simulink library "SimscapeCustomComponents_lib"  (R2025b)
settings: Solver=VariableStepAuto  StartTime=0.0  StopTime=10.0  RelTol=1e-3
undefined symbols (not defined in the file or in its folder): base, baseVdc, capacity, DiscIntNeverNeededParam, ee_sli_rtmsupport, filterInductance, freqeuncy, frequency, gcbh, gflInverter, gfmInverter, iMaxPU, Inertia, initialSOC, plantRating, solar, Ts, ups, Vac, windSystem, windTurbine
libraries: fl_lib x397, nesl_utility x171, eeGeneralControl x85, ee_lib x82, simulink x72, datacenter_lib x68, eeTransforms x38, slpidlib x24, buildingEnergy_lib x20, SimscapeFluids_lib x17, eeSinusoidalMeasurementV2 x8, eePwmGenerator x8
(part 21 of 24)

== system SimscapeCustomComponents_lib/Microgrid and Renewables/Sources/Solar Plant Integrated/Detailed/PV Plant & Controller/PV Plant/Converter/Switching ==
  mabc : Inport
  Add : Sum
  Constant1 : Constant
  Converter : ee_lib/Semiconductors & Converters/Converters/Converter (Three-Phase)  port_option=ee.enum.threePhasePort.composite  fidelity_option=ee.enum.converters.fidelity.detailed  device_type=ee.enum.converters.switchingdevice.ideal  showThermalPort=false  K=0  Vth=1 V  Vgt=1 V  Vgt_off=-1 V  Ih=1 A  Vf=0.8 V  Ron=0.001 Ohm  Rds=0.001 Ohm  Goff=1e-6 1/Ohm  Eon_scalar=22.86e-3 J  Eoff_scalar=17.14e-3 J  Eoff_natural_commutation=10e-3 J  Voff=300 V  Iout_scalar=600 A  onCurrentMeasDelay=0 s  useCurrentFromPreviousCycle=false  useVoltageFromPreviousCycle=false  diode_param=ee.enum.converters.protectiondiode.nodynamics  diode_Vf=0.01 V  diode_Ron=0.0001 Ohm  diode_Goff=1e-5 1/Ohm  diode_C=50 nF  diode_iRM=-235 A  diode_iF=300 A  diode_idot=-50 A/us  diode_trr_param=ee.enum.converters.diodetrr.trr_factor  diode_trr_factor=3  diode_trr=15 us  diode_Qrr=1500 s*uA  diode_rec_loss_model=ee.enum.diode.reverseRecoveryModel.fixed  diode_ErecVal=0 J  diode_scaleWithIandV=false  diode_ErecMat=zeros(2, 3) J  diode_TjrecVec=[298.15, 398.15] K  diode_IfrecVec=[.1, 1, 10] A  diode_IrecVal=10 A  diode_VrecVal=10 V  diode_tFilter=1 / 1000 / 100 s  thermal_network_parameterization=ee.enum.thermalNetworkTopology.external  Rth=[.08, .5] K/W  Rth_Cauer=[.08, .1, .5] K/W  Rth_Foster=[.08, .14, .22, .16] K/W  thermal_mass_parameterization=ee.enum.thermalNetwork.timeconstant  thermal_mass=[.01, .5] J/K  thermal_mass_Cauer=[.01, .1, .5] J/K  thermal_mass_Foster=[.001, .005, .05, .5] J/K  thermal_time_constant=[.001, .2] s  thermal_time_constant_Cauer=[.001, .1, .2] s  thermal_time_constant_Foster=[7e-05, .0007, .01, .08] s  thermal_mass_initial_temperatures=[25, 25] degC  thermal_mass_initial_temperatures_Cauer=[25, 25, 25] degC  junction_thermal_mass=0.01 J/K  Tvec_initial_Foster=[25, 25, 25, 25] degC  snubber_type=ee.enum.converters.snubber.exclude  Cs=1e-7 F  Rs=0.1 Ohm  Vce_loss=[0, 150, 300] V
  Demux : Demux  Outputs=3
  Demux1 : Demux  Outputs=3
  Gain : Gain  Gain=5
  Gain1 : Gain  Gain=0.5
  PWM Generator : eePwmGenerator/PWM Generator  CarrCount=Up  Tper=1/(fSw*1000)  Tdelay=0  Ts=1/(10*fSw*1000)
  Pulse Generation : Subsystem
  Rate Transition1 : RateTransition  OutPortSampleTime=1/(10*fSw*1000)
  Simulink-PS Converter{1..6} (6 alike) : nesl_utility/Simulink-PS Converter  PhysicalDomain=network_engine_domain  SubClassName=ps_input  LeftPortType=input  RightPortType=output  PseudoPeriodic=off  Frequencies=[]  NoiseDistribution=none  NoiseParameters=[]  Unit=1  AffineConversion=off  FilteringAndDerivatives=provide  SimscapeFilterOrder=1  InputFilterTimeConstant=0.001  UdotUserProvided=0
  Six-Pulse Gate Multiplexer : ee_lib/Semiconductors & Converters/Converters/Six-Pulse Gate Multiplexer  port_option=ee.enum.controlport.ps
  + : PMIOPort  Side=Left
  ~ : PMIOPort  Port=2  Side=Right
  - : PMIOPort  Port=3  Side=Left
  wires:
  [BH] -> Simulink-PS Converter4/1
  Pulse Generation/1(G1) -> Demux/1
  Pulse Generation/2(G2) -> Demux1/1
  Rate Transition1/1 -> PWM Generator/1
  Demux/1 -> [AH]
  Demux1/2 -> [BL]
  [AL] -> Simulink-PS Converter5/1
  [CH] -> Simulink-PS Converter2/1
  mabc/1 -> Add/1
  PWM Generator/1 -> Gain/1
  Gain/1 -> Pulse Generation/1(G)
  Add/1 -> Gain1/1
  Constant1/1 -> Add/2
  [CL] -> Simulink-PS Converter1/1
  Demux/2 -> [BH]
  Demux/3 -> [CH]
  Gain1/1 -> Rate Transition1/1
  Demux1/3 -> [CL]
  [AH] -> Simulink-PS Converter6/1
  [BL] -> Simulink-PS Converter3/1
  Demux1/1 -> [AL]
  connections:
  -/RConn1 -- Converter/RConn2
  +/RConn1 -- Converter/RConn1
  Six-Pulse Gate Multiplexer/LConn4 -- Simulink-PS Converter3/RConn1
  Six-Pulse Gate Multiplexer/LConn1 -- Simulink-PS Converter6/RConn1
  Six-Pulse Gate Multiplexer/RConn1 -- Converter/LConn1
  Six-Pulse Gate Multiplexer/LConn3 -- Simulink-PS Converter4/RConn1
  Simulink-PS Converter1/RConn1 -- Six-Pulse Gate Multiplexer/LConn6
  Simulink-PS Converter2/RConn1 -- Six-Pulse Gate Multiplexer/LConn5
  Six-Pulse Gate Multiplexer/LConn2 -- Simulink-PS Converter5/RConn1
  ~/RConn1 -- Converter/LConn2

== system SimscapeCustomComponents_lib/Microgrid and Renewables/Sources/Wind Plant Integrated/Detailed/Wind Turbine and Converters/Wind Controller/Machine Converter Control/Measurements ==
  iabc_sens : Inport
  w_sens : Inport  Port=2
  th_sens : Inport  Port=3
  Vdc_sens : Inport  Port=4
  2*pi : Constant  Value=2*pi  SampleTime=-1
  Math Function : Math  Operator=mod  SignedPower=on
  pole pairs : Gain  Gain=p
  "pole pairs " : Gain  Gain=p
  we : Outport  VectorParamsAs1DForOutWhenUnconnected=off
  iabc : Outport  Port=2  VectorParamsAs1DForOutWhenUnconnected=off
  theta : Outport  Port=3  VectorParamsAs1DForOutWhenUnconnected=off
  Vdc : Outport  Port=4  VectorParamsAs1DForOutWhenUnconnected=off
  wires:
  w_sens/1 -> pole pairs/1
  iabc_sens/1 -> iabc/1
  pole pairs/1 -> we/1
  2*pi/1 -> Math Function/2
  th_sens/1 -> "pole pairs "/1
  "pole pairs "/1 -> Math Function/1
  Vdc_sens/1 -> Vdc/1
  Math Function/1 -> theta/1

== system SimscapeCustomComponents_lib/Microgrid and Renewables/Sources/Wind Plant Integrated/Detailed/Wind Turbine and Converters/Wind Controller/Machine Converter Control/Power Controller ==
  windSpeed : Inport
  Derating Control : Subsystem
  Greater than : simulink/Logic and Bit Operations/Compare To Constant  relop=>  const=12  OutDataTypeStr=boolean
  Less than or equal to : simulink/Logic and Bit Operations/Compare To Constant  relop=<=  const=12  OutDataTypeStr=boolean
  Limiter Function Power Demand : Subsystem
  MPPT Control : Subsystem
  activePowerDemand : Outport
  wires:
  windSpeed/1 -> Greater than/1, Less than or equal to/1, MPPT Control/1(windSpeed)
  Less than or equal to/1 -> MPPT Control/Enable
  Greater than/1 -> Derating Control/Enable
  MPPT Control/1(activePowerDemand) -> Limiter Function Power Demand/1(activePowerDemandMPPT)
  Derating Control/1(activePowerDemand) -> Limiter Function Power Demand/2(activePowerDemandDerating)
  Limiter Function Power Demand/1(activePowerDemand) -> activePowerDemand/1

== system SimscapeCustomComponents_lib/Microgrid and Renewables/Sources/Wind Plant Integrated/Detailed/Wind Turbine and Converters/Wind Controller/Machine Converter Control/Subsystem ==
  note: LVRT Crowbar Control
  Vdc : Inport
  LVRT : Inport  Port=2
  Abs : Abs  SaturateOnIntegerOverflow=off
  Constant1 : Constant  Value=Vdc
  Product : Product
  Relay : Relay  OnSwitchValue=0.01001*Vdc  OffSwitchValue=0.01*Vdc
  Sum : Sum  Inputs=|+-
  Unit Delay1 : UnitDelay  SampleTime=-1
  Out1 : Outport
  wires:
  Constant1/1 -> Sum/1
  Vdc/1 -> Unit Delay1/1
  Sum/1 -> Product/1
  Abs/1 -> Relay/1
  Unit Delay1/1 -> Sum/2
  LVRT/1 -> Product/2
  Product/1 -> Abs/1
  Relay/1 -> Out1/1

== system SimscapeCustomComponents_lib/Microgrid and Renewables/Sources/Wind Plant Integrated/Detailed/Wind Turbine and Converters/Wind Controller/Wind Grid-side Converter Controller/Current_controller ==
  iWindd : Inport
  iq : Inport  Port=2
  id-ref : Inport  Port=3
  iqref : Inport  Port=4
  Vd : Inport  Port=5
  Vq : Inport  Port=6
  Constant4 : Constant  Value=0
  Gain1 : Gain  Gain=2*1*pi*frequency*inductance/baseImpedance
  Gain2 : Gain  Gain=2*1*pi*frequency*inductance/baseImpedance
  Mux1 : Mux  Inputs=3
  PI : Subsystem
  PI1 : Subsystem
  Sum1 : Sum  Inputs=|+-
  Sum3 : Sum  Inputs=|++-
  Sum4 : Sum  Inputs=|+++
  Sum5 : Sum  Inputs=|+-
  Refrence_mdq0 : Outport
  wires:
  PI/1(Out2) -> Sum3/2
  Sum3/1 -> Mux1/1, [Ed]
  Gain2/1 -> Sum3/3
  iWindd/1 -> Gain1/1, Sum1/2
  id-ref/1 -> Sum1/1
  Gain1/1 -> Sum4/3
  Vq/1 -> Sum4/2
  iq/1 -> Gain2/1, Sum5/2
  Sum1/1 -> PI/1(Input)
  Vd/1 -> Sum3/1
  Constant4/1 -> Mux1/3
  Sum5/1 -> PI1/1(Input)
  iqref/1 -> Sum5/1
  PI1/1(Out2) -> Sum4/1
  Sum4/1 -> Mux1/2, [Eq]
  Mux1/1 -> Refrence_mdq0/1  "m_dqo"

== system SimscapeCustomComponents_lib/Microgrid and Renewables/Sources/Wind Plant Integrated/Detailed/Wind Turbine and Converters/Wind Controller/Wind Grid-side Converter Controller/DC Bus Chopper control  ==
  note: LVRT Detection
  In1 : Inport
  Constant1 : Constant
  Constant2 : Constant  Value=0
  Switch : Switch  Criteria=u2 > Threshold  Threshold=0.9  SaturateOnIntegerOverflow=off  InputSameDT=off
  Unit Delay : UnitDelay  SampleTime=-1
  Out1 : Outport
  wires:
  Switch/1 -> Out1/1
  Constant1/1 -> Switch/3
  Constant2/1 -> Switch/1
  In1/1 -> Unit Delay/1
  Unit Delay/1 -> Switch/2

== system SimscapeCustomComponents_lib/Microgrid and Renewables/Sources/Wind Plant Integrated/Detailed/Wind Turbine and Converters/Wind Controller/Wind Grid-side Converter Controller/DC voltage controller & current reference ==
  note: Limiter
  note: iq_ref_generator
  note: id_ref_generator
  Q_ref : Inport
  Vmag : Inport  Port=2
  Wind_Mpp_vdc : Inport  Port=3
  Wind_vdc : Inport  Port=4
  lvrt.iq : Inport  Port=5
  Constant : Constant
  Constant1 : Constant  Value=iMaxPU
  Current limits : Subsystem
  Subsystem : Subsystem
  Subsystem1 : Subsystem
  Switch : Switch  Criteria=u2 > Threshold  SaturateOnIntegerOverflow=off  InputSameDT=off
  Unit Delay1 : UnitDelay  SampleTime=Ts
  Unit Delay3 : UnitDelay  SampleTime=Ts
  id_ref : Outport
  iq_ref : Outport  Port=2
  wires:
  Current limits/2(iubd) -> Subsystem1/3(id_ub)
  Subsystem/1(Out1) -> Unit Delay1/1, iq_ref/1
  Constant1/1 -> Current limits/1(Imax)
  Unit Delay1/1 -> Current limits/2(iqref)
  Subsystem1/1(Out1) -> id_ref/1, Unit Delay3/1
  Unit Delay3/1 -> Current limits/3(idref)
  Q_ref/1 -> Subsystem/4(Q_ref)
  Wind_Mpp_vdc/1 -> Subsystem1/1(Wind_Mpp_vdc)
  Wind_vdc/1 -> Subsystem1/2(Wind_vdc)
  Current limits/1(iubq) -> Subsystem/2(iq_ub)
  lvrt.iq/1 -> Subsystem/3(lvrt.iq)
  Vmag/1 -> Switch/1, Switch/2
  Switch/1 -> Subsystem/1(V_mag)
  Constant/1 -> Switch/3

== system SimscapeCustomComponents_lib/Microgrid and Renewables/Sources/Wind Plant Integrated/Detailed/Wind Turbine and Converters/Wind Plant/Back-to-Back Converters/Average ==
  Chopper : Inport
  SM_ref : Inport  Port=2
  Grid_ref : Inport  Port=3
  Capacitor : fl_lib/Electrical/Electrical Elements/Capacitor  c=capDC F  r=1e-1 Ohm  g=0 1/Ohm  i_specify=off  i_priority=None  i=0 A  i_nominal_specify=off  i_nominal_value=1  i_nominal_unit=A  v_specify=off  v_priority=None  v=0 V  v_nominal_specify=off  v_nominal_value=1  v_nominal_unit=V  vc_specify=on  vc_priority=High  vc=Vdc V  vc_nominal_specify=off  vc_nominal_value=1  vc_nominal_unit=V
  Electrical Reference : fl_lib/Electrical/Electrical Elements/Electrical Reference
  Electrical Reference1 : fl_lib/Electrical/Electrical Elements/Electrical Reference
  Electrical Reference2 : fl_lib/Electrical/Electrical Elements/Electrical Reference
  Grid Side Converter : ee_lib/Semiconductors & Converters/Converters/Average-Value Voltage Source Converter (Three-Phase)  port_option=ee.enum.threePhasePort.composite  frequency_option=ee.enum.converters.frequency.variable  input_option=ee.enum.converters.inputOption.ModWave  FRated=60 Hz  losses_parameterization=ee.enum.converters.losses.fixed  Pfixed=1 W  ks=0.01  kc1=1.7 V  kc2=0.01 Ohm  Ploss_vect=[100, 800, 1870, 3250, 4900] W  Irms_vect=[10, 100, 200, 300, 400] A  Vdc_nom=300 V  thermal_mass=30000 J/K  temperature_specify=off  temperature_priority=High  temperature=298.15 K  temperature_nominal_specify=off  temperature_nominal_value=1  temperature_nominal_unit=K
      settings: InternalSimscapePortConfiguration="{\"Bottom\":[],\"Left\":[{\"id\":\"ModWave\",\"label\":\"ModWave\",\"type\":\"input\"},{\"id\":\"N\",\"label\":\"~\",\"type\":\"foundation.electrical.three_phase\"}],\"Right\":[{\"id\":\"p\",\"label\":\"+\",\"type\":\"foundation.electrical.electrical\"},{\"id\":\"n\",\"label\":\"-\",\"type\":\"foundation.electrical.electrical\"}],\"Top\":[]}"
  Ideal Semiconductor Switch : ee_lib/Semiconductors & Converters/Ideal Semiconductor Switch  port_option=ee.enum.controlport.ps  Ron=0.001 Ohm  Goff=1e-6 1/Ohm  Vth=0.5 V  diode_param=ee.enum.converters.protectiondiode.none  diode_Vf=0.8 V  diode_Ron=0.001 Ohm  diode_Goff=1e-5 1/Ohm  diode_C=50e-9 F  diode_iRM=-235 A  diode_iF=300 A  diode_idot=-50 A/us  diode_trr_param=ee.enum.converters.diodetrr.trr_factor  diode_trr_factor=3  diode_trr=15 us  diode_Qrr=1500 s*uA
  Machine Side Converter : ee_lib/Semiconductors & Converters/Converters/Average-Value Voltage Source Converter (Three-Phase)  port_option=ee.enum.threePhasePort.composite  frequency_option=ee.enum.converters.frequency.variable  input_option=ee.enum.converters.inputOption.ModWave  FRated=60 Hz  losses_parameterization=ee.enum.converters.losses.fixed  Pfixed=1 W  ks=0.01  kc1=1.7 V  kc2=0.01 Ohm  Ploss_vect=[100, 800, 1870, 3250, 4900] W  Irms_vect=[10, 100, 200, 300, 400] A  Vdc_nom=300 V  thermal_mass=30000 J/K  temperature_specify=off  temperature_priority=High  temperature=298.15 K  temperature_nominal_specify=off  temperature_nominal_value=1  temperature_nominal_unit=K
      settings: InternalSimscapePortConfiguration="{\"Bottom\":[],\"Left\":[{\"id\":\"ModWave\",\"label\":\"ModWave\",\"type\":\"input\"},{\"id\":\"N\",\"label\":\"~\",\"type\":\"foundation.electrical.three_phase\"}],\"Right\":[{\"id\":\"p\",\"label\":\"+\",\"type\":\"foundation.electrical.electrical\"},{\"id\":\"n\",\"label\":\"-\",\"type\":\"foundation.electrical.electrical\"}],\"Top\":[]}"
  PS-Simulink Converter1 : nesl_utility/PS-Simulink Converter  PhysicalDomain=network_engine_domain  SubClassName=ps_output  LeftPortType=input  RightPortType=output  PseudoPeriodic=off  Frequencies=[]  VectorFormat=1-D array  Unit=V  AffineConversion=off
  Resistor : fl_lib/Electrical/Electrical Elements/Resistor  R=16 Ohm  i_specify=off  i_priority=None  i=0 A  i_nominal_specify=off  i_nominal_value=1  i_nominal_unit=A  v_specify=off  v_priority=None  v=0 V  v_nominal_specify=off  v_nominal_value=1  v_nominal_unit=V
  Scope : Scope
      settings: ActiveDisplayYMinimum=-0.125  ActiveDisplayYMaximum=1.125  DataLoggingVariableName=ScopeData11
  Simulink-PS Converter : nesl_utility/Simulink-PS Converter  PhysicalDomain=network_engine_domain  SubClassName=ps_input  LeftPortType=input  RightPortType=output  PseudoPeriodic=off  Frequencies=[]  NoiseDistribution=none  NoiseParameters=[]  Unit=1  AffineConversion=off  FilteringAndDerivatives=provide  SimscapeFilterOrder=1  InputFilterTimeConstant=0.001  UdotUserProvided=0
  Simulink-PS Converter2 : nesl_utility/Simulink-PS Converter  PhysicalDomain=network_engine_domain  SubClassName=ps_input  LeftPortType=input  RightPortType=output  PseudoPeriodic=off  Frequencies=[]  NoiseDistribution=none  NoiseParameters=[]  Unit=1  AffineConversion=off  FilteringAndDerivatives=provide  SimscapeFilterOrder=1  InputFilterTimeConstant=0.001  UdotUserProvided=0
  Simulink-PS Converter4 : nesl_utility/Simulink-PS Converter  PhysicalDomain=network_engine_domain  SubClassName=ps_input  LeftPortType=input  RightPortType=output  PseudoPeriodic=off  Frequencies=[]  NoiseDistribution=none  NoiseParameters=[]  Unit=1  AffineConversion=off  FilteringAndDerivatives=provide  SimscapeFilterOrder=1  InputFilterTimeConstant=0.001  UdotUserProvided=0
  Voltage Sensor : fl_lib/Electrical/Electrical Sensors/Voltage Sensor
  In : PMIOPort  Side=Left
  ~ : PMIOPort  Port=2  Side=Right
  Vdc : Outport
  wires:
  Grid_ref/1 -> Simulink-PS Converter4/1
  Chopper/1 -> Scope/1, Simulink-PS Converter2/1
  PS-Simulink Converter1/1 -> Vdc/1  "Vdc"
  SM_ref/1 -> Simulink-PS Converter/1
  connections:
  Electrical Reference/LConn1 -- Machine Side Converter/RConn2 -- Voltage Sensor/RConn2 -- Capacitor/RConn1
  Grid Side Converter/RConn1 -- Ideal Semiconductor Switch/RConn1 -- Capacitor/LConn1 -- Machine Side Converter/RConn1 -- Voltage Sensor/LConn1
  Electrical Reference2/LConn1 -- Grid Side Converter/RConn2
  PS-Simulink Converter1/LConn1 -- Voltage Sensor/RConn1
  ~/RConn1 -- Grid Side Converter/LConn2
  Resistor/LConn1 -- Ideal Semiconductor Switch/RConn2
  Grid Side Converter/LConn1 -- Simulink-PS Converter4/RConn1
  Electrical Reference1/LConn1 -- Resistor/RConn1
  Simulink-PS Converter2/RConn1 -- Ideal Semiconductor Switch/LConn1
  Machine Side Converter/LConn2 -- In/RConn1
  Simulink-PS Converter/RConn1 -- Machine Side Converter/LConn1

== system SimscapeCustomComponents_lib/Microgrid and Renewables/Sources/Wind Plant Integrated/Detailed/Wind Turbine and Converters/Wind Plant/Back-to-Back Converters/Switching ==
  Chopper : Inport
  SM_ref : Inport  Port=2
  Grid_ref : Inport  Port=3
  Capacitor : fl_lib/Electrical/Electrical Elements/Capacitor  c=capacitance F  r=1e-1 Ohm  g=0 1/Ohm  i_specify=off  i_priority=None  i=0 A  i_nominal_specify=off  i_nominal_value=1  i_nominal_unit=A  v_specify=off  v_priority=None  v=0 V  v_nominal_specify=off  v_nominal_value=1  v_nominal_unit=V  vc_specify=on  vc_priority=High  vc=baseVoltageDC V  vc_nominal_specify=off  vc_nominal_value=1  vc_nominal_unit=V
  Electrical Reference : fl_lib/Electrical/Electrical Elements/Electrical Reference
  Electrical Reference1 : fl_lib/Electrical/Electrical Elements/Electrical Reference
  Electrical Reference2 : fl_lib/Electrical/Electrical Elements/Electrical Reference
  Grid Side Converter : Subsystem
      settings: PortSchema="{\"entries\":[{\"content\":{\"sides\":[{\"content\":{\"connectorIds\":[\"LConn1\",\"LConn2\"]},\"type\":\"ConnectorPlacement.EquallySpacedRectSide\",\"uuid\":\"e32be008-cebd-46aa-ba62-c5c92b9b23e3\"},{\"content\":{\"connectorIds\":[\"In1\",\"RConn1\"],\"side\":\"RIGHT\"},\"type\":\"ConnectorPlacement.EquallySpacedRectSide\",\"uuid\":\"c483e451-04b5-4212-bdd1-c589ba5bea78\"},{\"content\":{\"side\":\"TOP\"},\"type\":\"ConnectorPlacement.EquallySpacedRectSide\",\"uuid\":\"824c135c-7e5f-4da0-a7de-e626b4bfa50d\"}]},\"type\":\"ConnectorPlacement.EquallySpacedConnector\",\"uuid\":\"5f81c72d-92ab-4525-91a6-193f769a7c86\"}],\"packageUris\":[\"http://schema.mathworks.com/mf0/Connector/R2020b\"],\"version\":\"1.0\"}"
  Ideal Semiconductor Switch : ee_lib/Semiconductors & Converters/Ideal Semiconductor Switch  port_option=ee.enum.controlport.ps  Ron=0.001 Ohm  Goff=1e-6 1/Ohm  Vth=0.5 V  diode_param=ee.enum.converters.protectiondiode.none  diode_Vf=0.8 V  diode_Ron=0.001 Ohm  diode_Goff=1e-5 1/Ohm  diode_C=50e-9 F  diode_iRM=-235 A  diode_iF=300 A  diode_idot=-50 A/us  diode_trr_param=ee.enum.converters.diodetrr.trr_factor  diode_trr_factor=3  diode_trr=15 us  diode_Qrr=1500 s*uA
  Machine Side Converter : Subsystem
      settings: PortSchema="{\"entries\":[{\"content\":{\"sides\":[{\"content\":{\"connectorIds\":[\"LConn1\",\"LConn2\"]},\"type\":\"ConnectorPlacement.EquallySpacedRectSide\",\"uuid\":\"e32be008-cebd-46aa-ba62-c5c92b9b23e3\"},{\"content\":{\"connectorIds\":[\"In1\",\"RConn1\"],\"side\":\"RIGHT\"},\"type\":\"ConnectorPlacement.EquallySpacedRectSide\",\"uuid\":\"c483e451-04b5-4212-bdd1-c589ba5bea78\"},{\"content\":{\"side\":\"TOP\"},\"type\":\"ConnectorPlacement.EquallySpacedRectSide\",\"uuid\":\"824c135c-7e5f-4da0-a7de-e626b4bfa50d\"}]},\"type\":\"ConnectorPlacement.EquallySpacedConnector\",\"uuid\":\"5f81c72d-92ab-4525-91a6-193f769a7c86\"}],\"packageUris\":[\"http://schema.mathworks.com/mf0/Connector/R2020b\"],\"version\":\"1.0\"}"
  PS-Simulink Converter1 : nesl_utility/PS-Simulink Converter  PhysicalDomain=network_engine_domain  SubClassName=ps_output  LeftPortType=input  RightPortType=output  PseudoPeriodic=off  Frequencies=[]  VectorFormat=1-D array  Unit=V  AffineConversion=off
  Resistor : fl_lib/Electrical/Electrical Elements/Resistor  R=16 Ohm  i_specify=off  i_priority=None  i=0 A  i_nominal_specify=off  i_nominal_value=1  i_nominal_unit=A  v_specify=off  v_priority=None  v=0 V  v_nominal_specify=off  v_nominal_value=1  v_nominal_unit=V
  Scope : Scope
      settings: ActiveDisplayYMinimum=-0.125  ActiveDisplayYMaximum=1.125  DataLoggingVariableName=ScopeData11
  Simulink-PS Converter2 : nesl_utility/Simulink-PS Converter  PhysicalDomain=network_engine_domain  SubClassName=ps_input  LeftPortType=input  RightPortType=output  PseudoPeriodic=off  Frequencies=[]  NoiseDistribution=none  NoiseParameters=[]  Unit=1  AffineConversion=off  FilteringAndDerivatives=provide  SimscapeFilterOrder=1  InputFilterTimeConstant=0.001  UdotUserProvided=0
  Voltage Sensor : fl_lib/Electrical/Electrical Sensors/Voltage Sensor
  In : PMIOPort  Side=Left
  ~ : PMIOPort  Port=2  Side=Right
  Vdc : Outport
  wires:
  SM_ref/1 -> Machine Side Converter/1(mabc)
  Grid_ref/1 -> Grid Side Converter/1(mabc)
  Chopper/1 -> Scope/1, Simulink-PS Converter2/1
  PS-Simulink Converter1/1 -> Vdc/1  "Vdc"
  connections:
  Machine Side Converter/LConn2 -- Voltage Sensor/RConn2 -- Capacitor/RConn1 -- Electrical Reference/LConn1
  Ideal Semiconductor Switch/RConn1 -- Grid Side Converter/LConn1 -- Capacitor/LConn1 -- Machine Side Converter/LConn1 -- Voltage Sensor/LConn1
  Grid Side Converter/LConn2 -- Electrical Reference2/LConn1
  PS-Simulink Converter1/LConn1 -- Voltage Sensor/RConn1
  ~/RConn1 -- Grid Side Converter/RConn1
  Resistor/LConn1 -- Ideal Semiconductor Switch/RConn2
  Electrical Reference1/LConn1 -- Resistor/RConn1
  Simulink-PS Converter2/RConn1 -- Ideal Semiconductor Switch/LConn1
  Machine Side Converter/RConn1 -- In/RConn1

== system SimscapeCustomComponents_lib/Microgrid and Renewables/Storage/BESS Integrated/Detailed/BESS Controller/Grid Following/Reference Current/Current limits ==
  Imax : Inport
  iqref : Inport  Port=2
  idref : Inport  Port=3
  Constant8 : Constant  Value=0
  Constant9 : Constant  Value=0
  Scope : Scope
      settings: ActiveDisplayYMinimum=-0.14399  ActiveDisplayYMaximum=1.29587  DataLoggingVariableName=ScopeData3
  Scope1 : Scope
      settings: ActiveDisplayYMinimum=-0.13655  ActiveDisplayYMaximum=1.22893  DataLoggingVariableName=ScopeData4
  Sqrt : Sqrt
  Sqrt1 : Sqrt
  Square{1..4} (4 alike) : Math  Operator=square
  Step2 : Step  Time=0.01  SampleTime=Ts
  Step3 : Step  Time=0.01  SampleTime=Ts
  Sum6 : Sum  Inputs=|+-
  Sum9 : Sum  Inputs=|+-
  Switch1 : Switch  Threshold=.01  SaturateOnIntegerOverflow=off  InputSameDT=off
  Switch2 : Switch  Threshold=.01  SaturateOnIntegerOverflow=off  InputSameDT=off
  iubq : Outport
  iubd : Outport  Port=2
  wires:
  Sum9/1 -> Switch2/1
  Step3/1 -> Switch2/2
  Step2/1 -> Switch1/2
  Switch2/1 -> Sqrt1/1
  Square1/1 -> Sum6/1
  Switch1/1 -> Sqrt/1
  iqref/1 -> Square2/1
  Square3/1 -> Sum9/1
  Sum6/1 -> Switch1/1
  Square2/1 -> Sum6/2
  Constant8/1 -> Switch1/3
  Square4/1 -> Sum9/2
  Constant9/1 -> Switch2/3
  Sqrt/1 -> Scope/1, iubd/1
  Imax/1 -> Square3/1, Square1/1
  Sqrt1/1 -> Scope1/1, iubq/1
  idref/1 -> Square4/1

== system SimscapeCustomComponents_lib/Microgrid and Renewables/Storage/BESS Integrated/Detailed/BESS Controller/Grid Following/Reference Current/Refernce id generation ==
  V_mag : Inport
  del f : Inport  Port=2
  ubid : Inport  Port=3
  PRef : Inport  Port=4
  Divide : Product  Inputs=/*
  Gain6 : Gain  Gain=-1
  P/Q Priority : Switch  Criteria=u2 ~= 0  SaturateOnIntegerOverflow=off  InputSameDT=off
  Priority Mode : Constant  Value=P-2
  Saturation Dynamic2 : simulink/Discontinuities/Saturation Dynamic  OutMin=[]  OutMax=[]  OutDataTypeStr=Inherit: Same as second input  OutDataType=fixdt(1, 16)  OutScaling=2^-10  DoSatur=off
  Saturation1 : Saturate  UpperLimit=Imax  LowerLimit=-Imax
  Scope : Scope
      settings: ActiveDisplayYMinimum=-1  ActiveDisplayYMaximum=1
  Scope1 : Scope
      settings: ActiveDisplayYMinimum=-0.68622  ActiveDisplayYMaximum=0.07625  DataLoggingVariableName=ScopeData2
  Sum : Sum  Inputs=|++
  droop m_p : Gain  Gain=mp/MVA
  ubid1 : InportShadow  Port=3
  id_ref : Outport
  wires:
  droop m_p/1 -> Sum/1
  Sum/1 -> Divide/2
  ubid/1 -> Saturation Dynamic2/1
  Gain6/1 -> Saturation Dynamic2/3
  Saturation Dynamic2/1 -> Scope1/1, P/Q Priority/3
  PRef/1 -> Sum/2
  Priority Mode/1 -> P/Q Priority/2
  Saturation1/1 -> P/Q Priority/1
  ubid1/1 -> Gain6/1
  P/Q Priority/1 -> Scope/1, id_ref/1
  V_mag/1 -> Divide/1
  Divide/1 -> Saturation1/1, Saturation Dynamic2/2
  del f/1 -> droop m_p/1

== system SimscapeCustomComponents_lib/Microgrid and Renewables/Storage/BESS Integrated/Detailed/BESS Controller/Grid Following/Reference Current/Refernce iq generation ==
  ubiq : Inport
  V_ref : Inport  Port=2
  V_mag : Inport  Port=3
  LVRT_iq : Inport  Port=4
  Q_ref : Inport  Port=5
  Divide1 : Product  Inputs=*/
  Gain : Gain  Gain=-1
  Gain1 : Gain  Gain=-1
  Gain7 : Gain  Gain=-1
  LVRT Priority : Switch  Threshold=.9  SaturateOnIntegerOverflow=off  InputSameDT=off
  P/Q Priority : Switch  Criteria=u2 ~= 0  SaturateOnIntegerOverflow=off  InputSameDT=off
  Priority Mode : Constant  Value=P-2
  Saturation Dynamic : simulink/Discontinuities/Saturation Dynamic  OutMin=[]  OutMax=[]  OutDataTypeStr=Inherit: Same as second input  OutDataType=fixdt(1, 16)  OutScaling=2^-10  DoSatur=off
  Saturation2 : Saturate  UpperLimit=1  LowerLimit=-1
  Saturation3 : Saturate  UpperLimit=Imax  LowerLimit=-Imax
  Sum : Sum  Inputs=|++
  Sum1 : Sum  Inputs=|-+
  droop m_v : Gain  Gain=mv
  ubiq1 : InportShadow
  iq_ref : Outport
  wires:
  LVRT Priority/1 -> Gain/1
  Sum1/1 -> droop m_v/1
  P/Q Priority/1 -> LVRT Priority/1
  Gain1/1 -> LVRT Priority/3
  ubiq/1 -> Saturation Dynamic/1
  Saturation2/1 -> Gain1/1
  Saturation3/1 -> P/Q Priority/3
  Priority Mode/1 -> P/Q Priority/2
  Divide1/1 -> Saturation Dynamic/2, Saturation3/1
  Saturation Dynamic/1 -> P/Q Priority/1
  Gain7/1 -> Saturation Dynamic/3
  V_ref/1 -> Sum1/1
  LVRT_iq/1 -> Saturation2/1
  ubiq1/1 -> Gain7/1
  droop m_v/1 -> Sum/2
  Sum/1 -> Divide1/1
  Q_ref/1 -> Sum/1
  V_mag/1 -> LVRT Priority/2, Divide1/2, Sum1/2
  Gain/1 -> iq_ref/1

== system SimscapeCustomComponents_lib/Microgrid and Renewables/Storage/BESS Integrated/Detailed/BESS Controller/Grid Forming/Current Limiting/CurrentLimitingMethod ==
  Igd : Inport
  Igq : Inport  Port=2
  currentLimitAndVirtual : Subsystem  VariantControl=both
  currentSaturation : Subsystem  VariantControl=ctSat
  virtualImpedance : Subsystem  VariantControl=virimp
  delVd : Outport
  delVq : Outport  Port=2
  Idmax : Outport  Port=3
  Iqmax : Outport  Port=4

== system SimscapeCustomComponents_lib/Microgrid and Renewables/Storage/BESS Integrated/Detailed/BESS Controller/Grid Forming/Grid Voltage Reactive Power Support/Modifying Active Power Reference ==
  PrefInput : Inport
  Vd : Inport  Port=2
  Igd : Inport  Port=3
  Igq : Inport  Port=4
  AND : Logic  IconShape=distinctive  AllPortsSameDT=off  OutDataTypeStr=boolean
  Abs : Abs  SaturateOnIntegerOverflow=off
  Compare To Constant : simulink/Logic and Bit Operations/Compare To Constant  relop=>=  const=0.95  OutDataTypeStr=boolean
  Computing New Active Power Ref : Subsystem
  Math Function1 : Math  Operator=hypot
  Power Sign : Signum
  Product : Product
  Relay : Relay  OnSwitchValue=40%maxVICurrentLimit*0.96  OffSwitchValue=1
  Scope : Scope
  Scope1 : Scope
  Scope2 : Scope
  Switch : Switch  Criteria=u2 > Threshold  SaturateOnIntegerOverflow=off  InputSameDT=off
  Pref : Outport
  wires:
  Computing New Active Power Ref/1(Pref) -> Switch/1, Scope/1
  Math Function1/1 -> Scope2/1, Relay/1  "Is"
  Vd/1 -> Computing New Active Power Ref/2(Vd), Compare To Constant/1
  PrefInput/1 -> Power Sign/1, Switch/3
  Igd/1 -> Math Function1/2
  Igq/1 -> Computing New Active Power Ref/1(Iq), Math Function1/1
  Switch/1 -> Abs/1
  Abs/1 -> Product/1
  Power Sign/1 -> Product/2
  Product/1 -> Pref/1
  Relay/1 -> Scope1/1, AND/2
  AND/1 -> Switch/2
  Compare To Constant/1 -> AND/1

== system SimscapeCustomComponents_lib/Microgrid and Renewables/Storage/BESS Integrated/Detailed/BESS Controller/Grid Forming/Grid Voltage Reactive Power Support/Modifying Reactive Power Reference ==
  Vgd : Inport
  Vgq : Inport  Port=2
  Qref : Inport  Port=3
  Pref : Inport  Port=4
  Changing the Power Reference : Subsystem
  Hysteresis : Subsystem
  Math Function : Math  Operator=hypot
  Merge : Merge
  Merge1 : Merge
  NOT : Logic  Operator=NOT  IconShape=distinctive  AllPortsSameDT=off  OutDataTypeStr=boolean
  Not Altering the Power Reference : Subsystem
  Scope : Scope
  PrefNew : Outport
  QrefNew : Outport  Port=2
  wires:
  Vgd/1 -> [Vd], Math Function/1
  Not Altering the Power Reference/2(Qrefv) -> Merge1/2
  Math Function/1 -> Hysteresis/1(Vs), [Vs]
  [Vs] -> Changing the Power Reference/1(Vs)
  Not Altering the Power Reference/1(Prefv) -> Merge/2
  Changing the Power Reference/1(Prefv) -> Merge/1
  NOT/1 -> Not Altering the Power Reference/Enable
  Qref/1 -> Not Altering the Power Reference/2(Qref), [Qref]
  Hysteresis/1(LVFlag) -> Scope/1, Changing the Power Reference/Enable, NOT/1
  [Vd] -> Changing the Power Reference/2(Vd)
  Changing the Power Reference/2(Qrefv) -> Merge1/1
  Vgq/1 -> Math Function/2
  Pref/1 -> Not Altering the Power Reference/1(Pref), [Pref]
  Merge1/1 -> QrefNew/1
  Merge/1 -> PrefNew/1
  [Pref] -> Changing the Power Reference/3(Pref)
  [Qref] -> Changing the Power Reference/4(Qref)

== system SimscapeCustomComponents_lib/Microgrid and Renewables/Storage/BESS Integrated/Detailed/BESS Controller/Grid Forming/Measurement/Frequency Measurement ==
  Vabc : Inport
  Convert To PU : Gain  Gain=1/powerFreq
  Frequency Measurement : Subsystem  TreatAsAtomicUnit=on  SystemSampleTime=sampleTime  mask{initialFrequency=powerFreq, sampleTime=activePowerSampleTime}
      mask prompts: initialFrequency "Initial frequency in Hz"; sampleTime "Sample time in sec"
      mask DialogControl Container7 Prompt: General
  Low-Pass Filter : eeGeneralControl/Low-Pass Filter (Discrete or Continuous)  K=1  T=freqMeasTimeConst  B=inf  A=-inf  init_option=Inherited from block input  x0=0  Ts=-1
  freq : Outport
  wires:
  Low-Pass Filter/1 -> Convert To PU/1  "Freq"
  Frequency Measurement/1(Freq) -> Low-Pass Filter/1
  Convert To PU/1 -> freq/1
  Vabc/1 -> Frequency Measurement/1(abc)

== system SimscapeCustomComponents_lib/Microgrid and Renewables/Storage/BESS Integrated/Detailed/BESS Controller/Grid Forming/Measurement/abc2dq ==
  Igabc : Inport
  Angle : Inport  Port=2
  Vgabc : Inport  Port=3
  Supply Current to dq : Subsystem
  Supply Voltage  to dq1 : Subsystem
  Vgd : Outport
  Vgq : Outport  Port=2
  Igd : Outport  Port=3
  Igq : Outport  Port=4
  wires:
  Angle/1 -> Supply Voltage  to dq1/1(Angle), Supply Current to dq/2(Angle)
  Vgabc/1 -> Supply Voltage  to dq1/2(abc)
  Igabc/1 -> Supply Current to dq/1(abc)
  Supply Current to dq/1(Igd) -> Igd/1  "Id"
  Supply Current to dq/2(Igq) -> Igq/1  "Iq"
  Supply Voltage  to dq1/1(Vgd) -> Vgd/1  "Vgd"
  Supply Voltage  to dq1/2(Vgq) -> Vgq/1  "Vgq"

== system SimscapeCustomComponents_lib/Microgrid and Renewables/Storage/BESS Integrated/Detailed/BESS Controller/Grid Forming/Power Control/ActivePowerControl ==
  Pref : Inport
  Pmeas : Inport  Port=2
  fref : Inport  Port=3
  cntrlflag : Inport  Port=4
  fgrid : Inport  Port=5
  droopControl : Subsystem  VariantControl=droop
  vsmControl : Subsystem  VariantControl=vsm
  Theta : Outport
  w : Outport  Port=2

== system SimscapeCustomComponents_lib/Microgrid and Renewables/Storage/BESS Integrated/Detailed/BESS Controller/Grid Forming/Power Control/ReactiveControl ==
  note: Vs-delV
  CntrlFlag : Inport
  Qref : Inport  Port=2
  Qmeas : Inport  Port=3
  Vgdmeas : Inport  Port=4
  Vref : Inport  Port=5
  Constant2 : Constant  Value=0
  Saturation1 : Saturate  UpperLimit=(dcBusVoltage/2)/(sqrt(2/3)*girdLineVoltage)  LowerLimit=-(dcBusVoltage/2)/(sqrt(2/3)*girdLineVoltage)
  Scope : Scope
      settings: ActiveDisplayYMinimum=0.99958  ActiveDisplayYMaximum=1.0007  DataLoggingVariableName=ScopeData20
  Voltage  Reference Selection : Subsystem
  Vmd : Outport
  Vmq : Outport  Port=2
  wires:
  Voltage  Reference Selection/1(Vd) -> Saturation1/1  "Q"
  Constant2/1 -> Vmq/1
  Saturation1/1 -> Scope/1, Vmd/1
  CntrlFlag/1 -> Voltage  Reference Selection/1(cntrlflag)
  Qref/1 -> Voltage  Reference Selection/2(Qref)
  Qmeas/1 -> Voltage  Reference Selection/3(Qmeas)
  Vref/1 -> Voltage  Reference Selection/4(Vref)
  Vgdmeas/1 -> Voltage  Reference Selection/5(Vgdmeas)

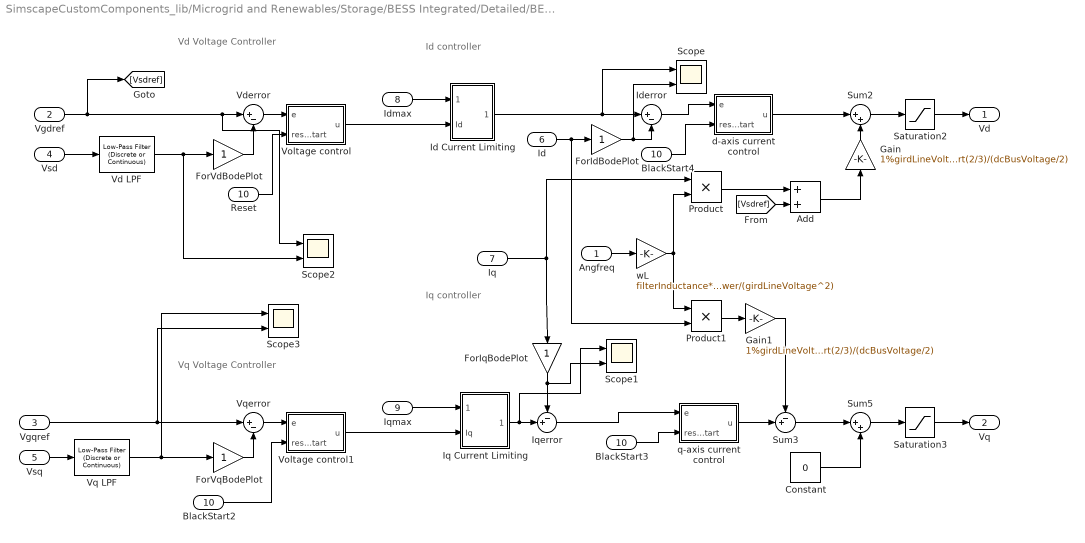
== system SimscapeCustomComponents_lib/Microgrid and Renewables/Storage/BESS Integrated/Detailed/BESS Controller/Grid Forming/VoltageCurrentControl/Controller ==
  note: Id controller
  note: Vd Voltage Controller
  note: Iq controller
  note: Vq Voltage Controller
  Angfreq : Inport
  Vgdref : Inport  Port=2
  Vgqref : Inport  Port=3
  Vsd : Inport  Port=4
  Vsq : Inport  Port=5
  Id : Inport  Port=6
  Iq : Inport  Port=7
  Idmax : Inport  Port=8
  Iqmax : Inport  Port=9
  Reset : Inport  Port=10
  Add : Sum
  BlackStart2 : InportShadow  Port=10
  BlackStart3 : InportShadow  Port=10
  BlackStart4 : InportShadow  Port=10
  Constant : Constant  Value=0  SampleTime=currentControlTs
  ForIdBodePlot : Gain
  ForIqBodePlot : Gain
  ForVdBodePlot : Gain
  ForVqBodePlot : Gain
  Gain : Gain  Gain=1%girdLineVoltage*sqrt(2/3)/(dcBusVoltage/2)
  Gain1 : Gain  Gain=1%girdLineVoltage*sqrt(2/3)/(dcBusVoltage/2)
  Id Current Limiting : Subsystem
  Iderror : Sum  Inputs=|+-
  Iq Current Limiting : Subsystem
  Iqerror : Sum  Inputs=-+|
  Product : Product
  Product1 : Product
  Saturation2 : Saturate  UpperLimit=4  LowerLimit=-3
  Saturation3 : Saturate  UpperLimit=3  LowerLimit=-3
  Scope{,1..3} (4 alike) : Scope  NumInputPorts=2
      Scope settings: ActiveDisplayYMinimum=-0.33488  ActiveDisplayYMaximum=2.03721
      Scope2 settings: ActiveDisplayYMinimum=-0.14129  ActiveDisplayYMaximum=1.2716
  Sum2 : Sum  Inputs=|++
  Sum3 : Sum  Inputs=-+|
  Sum5 : Sum  Inputs=|++
  Vd LPF : eeGeneralControl/Low-Pass Filter (Discrete or Continuous)  K=1  T=vdvqLPFTimeConst  B=inf  A=-inf  init_option=Specify as parameter  x0=0  Ts=voltControlTs
  Vderror : Sum  Inputs=|+-
  Voltage control : Subsystem
  Voltage control1 : Subsystem
  Vq LPF : eeGeneralControl/Low-Pass Filter (Discrete or Continuous)  K=1  T=vdvqLPFTimeConst  B=inf  A=-inf  init_option=Inherited from block input  x0=0  Ts=voltControlTs
  Vqerror : Sum  Inputs=|+-
  d-axis current control : Subsystem
  q-axis current control : Subsystem
  wL : Gain  Gain=filterInductance*power/(girdLineVoltage^2)
  Vd : Outport  VectorParamsAs1DForOutWhenUnconnected=off
  Vq : Outport  Port=2  VectorParamsAs1DForOutWhenUnconnected=off
  wires:
  Iqerror/1 -> q-axis current control/1(e)
  wL/1 -> Product1/1, Product/2
  Iq/1 -> ForIqBodePlot/1, Product/1
  Angfreq/1 -> wL/1
  Constant/1 -> Sum5/2
  Iderror/1 -> d-axis current control/1(e)
  Saturation3/1 -> Vq/1
  Saturation2/1 -> Vd/1
  Product1/1 -> Gain1/1
  Product/1 -> Add/1
  d-axis current control/1(u) -> Sum2/1
  Sum2/1 -> Saturation2/1
  q-axis current control/1(u) -> Sum3/2
  Sum3/1 -> Sum5/1
  Sum5/1 -> Saturation3/1
  Vsq/1 -> Vq LPF/1
  Id/1 -> Product1/2, ForIdBodePlot/1
  Vderror/1 -> Voltage control/1(e)
  Iqmax/1 -> Iq Current Limiting/1(Imax)
  Vgqref/1 -> Scope3/2, Vqerror/1
  Vqerror/1 -> Voltage control1/1(e)
  Gain1/1 -> Sum3/1
  [Vsdref] -> Add/2
  Add/1 -> Gain/1
  Gain/1 -> Sum2/2
  Voltage control/1(u) -> Id Current Limiting/2(Id)
  Idmax/1 -> Id Current Limiting/1(Imax)
  Iq Current Limiting/1(Iqref) -> Scope1/1, Iqerror/2
  Voltage control1/1(u) -> Iq Current Limiting/2(Iq)
  Vsd/1 -> Vd LPF/1
  ForVdBodePlot/1 -> Vderror/2
  ForVqBodePlot/1 -> Vqerror/2
  ForIdBodePlot/1 -> Scope/2, Iderror/2
  ForIqBodePlot/1 -> Scope1/2, Iqerror/1
  Id Current Limiting/1(Idref) -> Scope/1, Iderror/1
  Vd LPF/1 -> Scope2/2, ForVdBodePlot/1
  Vq LPF/1 -> Scope3/1, ForVqBodePlot/1
  Reset/1 -> Voltage control/2(resetBlackStart)
  BlackStart2/1 -> Voltage control1/2(resetBlackStart)
  BlackStart3/1 -> q-axis current control/2(resetBlackStart)
  BlackStart4/1 -> d-axis current control/2(resetBlackStart)
  Vgdref/1 -> Scope2/1, Vderror/1, [Vsdref]

== system SimscapeCustomComponents_lib/Microgrid and Renewables/Storage/BESS Integrated/Detailed/BESS Controller/Grid Forming/VoltageCurrentControl/Modulation Signal ==
  Vd : Inport
  Vq : Inport  Port=2
  Angle : Inport  Port=3
  Constant : Constant  Value=0
  Inverse Park Transform : eeTransforms/Inverse Park Transform  AxisAlignment=D-axis  PowerInvariant=off
  Mux1 : Mux  Inputs=3
  Saturation2 : Saturate  UpperLimit=1  LowerLimit=-1
  Scope : Scope  NumInputPorts=2
      settings: DataLoggingVariableName=ScopeData9
  Scope1 : Scope
  mabc : Outport  VectorParamsAs1DForOutWhenUnconnected=off
  wires:
  Inverse Park Transform/1 -> Saturation2/1
  Mux1/1 -> Inverse Park Transform/1
  Angle/1 -> Scope1/1, Inverse Park Transform/2
  Saturation2/1 -> mabc/1
  Constant/1 -> Mux1/3
  Vd/1 -> Scope/1, Mux1/1
  Vq/1 -> Scope/2, Mux1/2

== system SimscapeCustomComponents_lib/Microgrid and Renewables/Storage/BESS Integrated/Detailed/BESS Plant/Converter/Switching/Pulse Generation ==
  G : Inport
  Constant : Constant  Value=5
  Subtract : Sum  Inputs=-+
  G1 : Outport  VectorParamsAs1DForOutWhenUnconnected=off
  G2 : Outport  Port=2  VectorParamsAs1DForOutWhenUnconnected=off
  wires:
  Subtract/1 -> G2/1
  Constant/1 -> Subtract/2
  G/1 -> G1/1, Subtract/1

== system SimscapeCustomComponents_lib/Microgrid and Renewables/Control/BESS/Grid Forming Control/Current Limiting/CurrentLimitingMethod/currentLimitAndVirtual/Current Saturation/Compare ==
  u : Inport
  Compare To Zero : simulink/Logic and Bit Operations/Compare To Zero  relop=<=  OutDataTypeStr=boolean
  Data Type Conversion : DataTypeConversion  SaturateOnIntegerOverflow=off  RndMeth=Floor
  Out1 : Outport
  wires:
  Compare To Zero/1 -> Data Type Conversion/1
  u/1 -> Compare To Zero/1
  Data Type Conversion/1 -> Out1/1

== system SimscapeCustomComponents_lib/Microgrid and Renewables/Control/BESS/Grid Forming Control/Current Limiting/CurrentLimitingMethod/currentLimitAndVirtual/Current Saturation/If Action Subsystem ==
  Is : Inport
  Isd : Inport  Port=2
  Isq : Inport  Port=3
  maxI : Inport  Port=4
  Action Port : ActionPort
  Divide : Product  Inputs=*/
  Product : Product
  Product1 : Product
  Idmax : Outport
  Iqmax : Outport  Port=2
  wires:
  maxI/1 -> Divide/1
  Is/1 -> Divide/2
  Divide/1 -> Product1/2, Product/1
  Isd/1 -> Product1/1
  Isq/1 -> Product/2
  Product1/1 -> Idmax/1
  Product/1 -> Iqmax/1

== system SimscapeCustomComponents_lib/Microgrid and Renewables/Control/BESS/Grid Forming Control/Current Limiting/CurrentLimitingMethod/currentLimitAndVirtual/Current Saturation/If Action Subsystem1 ==
  Action Port : ActionPort
  Constant3 : Constant  Value=0
  Constant4 : Constant  Value=0
  Idmax : Outport
  Iqmax : Outport  Port=2
  wires:
  Constant4/1 -> Iqmax/1
  Constant3/1 -> Idmax/1

== system SimscapeCustomComponents_lib/Microgrid and Renewables/Control/BESS/Grid Forming Control/Measurement/Frequency Measurement/Frequency Measurement/If Action Subsystem/Frequency estimation ==
  sk : Inport
  sk-1 : Inport  Port=2
  k : Inport  Port=3
  k-1 : Inport  Port=4
  Trigger : TriggerPort  VariantControl=(inherit)  InitialTriggerSignalState=positive
  Add1 : Sum  Inputs=+-  OutDataTypeStr=double  AccumDataTypeStr=double  RndMeth=Convergent
  Add2 : Sum
  Constant : Constant
  Delay : Delay  DelayLength=1
  Delay1 : Delay  DelayLength=1
  Divide : Product  Inputs=*/  RndMeth=Ceiling
  Gain : Gain  Gain=2  ParamDataTypeStr=double  RndMeth=Convergent
  Gain2 : Gain  Gain=0.5
  MATLAB Function : MATLAB Function  TreatAsAtomicUnit=on
  f : Outport
  wires:
  Add1/1 -> Gain/1
  Constant/1 -> Divide/1
  Gain/1 -> Divide/2
  MATLAB Function/1(x) -> Delay/1, Add1/1  "x1-y1/slope"
  Divide/1 -> Add2/1, Delay1/1
  Delay1/1 -> Add2/2
  Add2/1 -> Gain2/1
  Gain2/1 -> f/1
  Delay/1 -> Add1/2
  k/1 -> MATLAB Function/3(x1)
  k-1/1 -> MATLAB Function/4(x2)  "x1"
  sk/1 -> MATLAB Function/1(y1)
  sk-1/1 -> MATLAB Function/2(y2)

== system SimscapeCustomComponents_lib/Microgrid and Renewables/Control/BESS/Grid Forming Control/Power Control/ActivePowerControl/vsmControl/Damping Frequency/ConstantFreqReference ==
  fref : Inport
  Constant1 : Constant
  Terminator : Terminator
  fmeas : Outport
  wires:
  Constant1/1 -> fmeas/1
  fref/1 -> Terminator/1

== system SimscapeCustomComponents_lib/Microgrid and Renewables/Control/BESS/Grid Forming Control/Power Control/ActivePowerControl/vsmControl/Damping Frequency/WithFrequencyMeasurement ==
  fref : Inport
  fmeas : Outport
  wires:
  fref/1 -> fmeas/1

== system SimscapeCustomComponents_lib/Microgrid and Renewables/Control/BESS/Grid Forming Control/Power Control/ActivePowerControl/vsmControl/Power Reference Selection/If Action Subsystem ==
  note: Frequency difference power
  Pref : Inport
  Wsm : Inport  Port=2
  Action Port : ActionPort
  Constant : Constant
  Gain6 : Gain  Gain=vsmFreqDroop
  Sum : Sum  Inputs=|+-
  Sum3 : Sum  Inputs=++|
  Power : Outport
  wires:
  Gain6/1 -> Sum3/2
  Pref/1 -> Sum3/1  "Reference power"
  Wsm/1 -> Sum/2
  Sum/1 -> Gain6/1
  Constant/1 -> Sum/1
  Sum3/1 -> Power/1

== system SimscapeCustomComponents_lib/Microgrid and Renewables/Control/BESS/Grid Forming Control/Power Control/ActivePowerControl/vsmControl/Power Reference Selection/If Action Subsystem1 ==
  note: Frequency difference power
  fref : Inport
  Wsm : Inport  Port=2
  Action Port : ActionPort
  Gain6 : Gain  Gain=vsmFreqDroop
  Scope : Scope
      settings: ActiveDisplayYMinimum=0.99966  ActiveDisplayYMaximum=1.00057  DataLoggingVariableName=ScopeData14
  Scope1 : Scope
      settings: DataLoggingVariableName=ScopeData15
  Sum : Sum  Inputs=|+-
  Power : Outport
  wires:
  Wsm/1 -> Scope/1, Sum/2
  Sum/1 -> Gain6/1
  fref/1 -> Sum/1
  Gain6/1 -> Scope1/1, Power/1

== system SimscapeCustomComponents_lib/Microgrid and Renewables/Control/Renewables/Wind Controller/Wind Grid-side Converter Controller/DC voltage controller & current reference/Subsystem1/V_dc_Controller1/PI ==
  Input : Inport
  Discrete-Time Integrator : DiscreteIntegrator  gainval=Ki_dc  SampleTime=Ts  ICPrevOutput=DiscIntNeverNeededParam  ICPrevScaledInput=DiscIntNeverNeededParam
  Gain1 : Gain  Gain=Kp_dc
  Sum1 : Sum  Inputs=|++
  Unit Delay : UnitDelay  SampleTime=Ts
  Out2 : Outport
  wires:
  Discrete-Time Integrator/1 -> Sum1/1
  Sum1/1 -> Out2/1
  Unit Delay/1 -> Sum1/2
  Gain1/1 -> Unit Delay/1
  Input/1 -> Gain1/1, Discrete-Time Integrator/1
